simulink model "test1"  (R2023b)
settings: Solver=VariableStepAuto  StartTime=0.0  StopTime=100  RelTol=1e-3
values from neighbouring files (symbols this model uses):
  v_min_controllable = 20    [para_sim1dot0.mat]    (also in para_sim1dot1.mat; para_sim1dot2.mat; para_sim1dot3.mat; para_sim1dot4.mat)
libraries: robotcorelib x2, sharedtransform x1, simulink x1
settings Model: Creator=Zian Liu  LastModifiedBy=Zian Liu

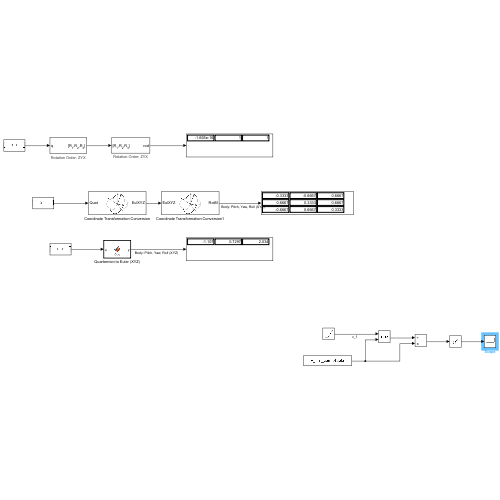
[thumbnail: Simulink's stored preview of the top-level diagram]
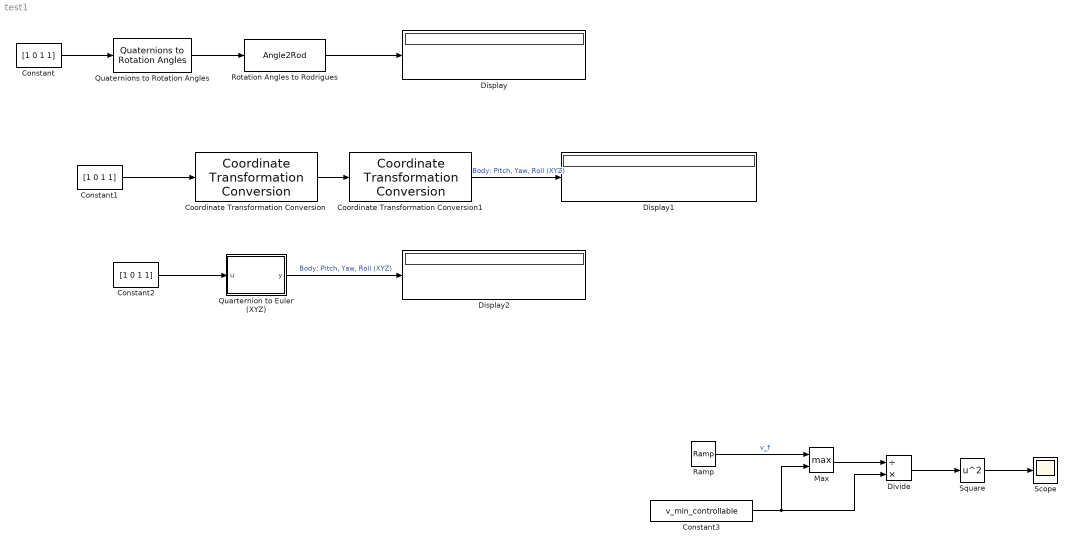
== system test1 ==
  Constant : Constant  Value=[1 0 1 1]
  Constant1 : Constant  Value=[1 0 1 1]
  Constant2 : Constant  Value=[1 0 1 1]  VectorParams1D=off
  Constant3 : Constant  Value=v_min_controllable
  Coordinate Transformation Conversion : robotcorelib/Coordinate Transformation Conversion  InputRepresentation=Quaternion  InputEulerSequence=ZYX  ShowTrVecInputPort=on  OutputRepresentation=Euler Angles  OutputEulerSequence=XYZ  ShowTrVecOutputPort=on  SimulateUsing=Interpreted execution
      settings: LibrarySourceBlock=uavutilslib/Coordinate Transformation Conversion
  Coordinate Transformation Conversion1 : robotcorelib/Coordinate Transformation Conversion  InputRepresentation=Euler Angles  InputEulerSequence=XYZ  ShowTrVecInputPort=on  OutputRepresentation=Rotation Matrix  OutputEulerSequence=XYZ  ShowTrVecOutputPort=on  SimulateUsing=Interpreted execution
      settings: LibrarySourceBlock=uavutilslib/Coordinate Transformation Conversion
  Display : Display
  Display1 : Display
  Display2 : Display
  Divide : Product  Inputs=/*
  Max : MinMax  Function=max  Inputs=2
  Quarternion to Euler (XYZ) : MATLAB Function  TreatAsAtomicUnit=on
  Quaternions to Rotation Angles : sharedtransform/Quaternions to Rotation Angles  rotationOrder=ZYX  aMode=aMode
  Ramp : simulink/Sources/Ramp  slope=1  start=0  InitialOutput=0
  Rotation Angles to Rodrigues : Angle2Rod
      settings: AttributesFormatString=Rotation Order: %<rotationOrder>
  Scope : Scope
  Square : Math  Operator=square
  wires:
  Constant/1 -> Quaternions to Rotation Angles/1
  Rotation Angles to Rodrigues/1 -> Display/1
  Quaternions to Rotation Angles/1 -> Rotation Angles to Rodrigues/1
  Constant1/1 -> Coordinate Transformation Conversion/1
  Coordinate Transformation Conversion/1 -> Coordinate Transformation Conversion1/1
  Constant2/1 -> Quarternion to Euler (XYZ)/1(u)
  Quarternion to Euler (XYZ)/1(y) -> Display2/1  "Body: Pitch, Yaw, Roll (XYZ)"
  Coordinate Transformation Conversion1/1 -> Display1/1  "Body: Pitch, Yaw, Roll (XYZ)"
  Constant3/1 -> Max/2, Divide/2
  Ramp/1 -> Max/1  "v_f"
  Divide/1 -> Square/1
  Max/1 -> Divide/1
  Square/1 -> Scope/1

== matlab function test1/Quarternion to Euler (XYZ) ==
  data: u input; y output
function y = fcn(u)
quatnormalize(u)
y = quat2eul(u, 'XYZ')
